simulink model "microphone_PDM"  (R2016b)
settings: Solver=ode5  StartTime=0.0  StopTime=2*pi*200000/2.4e6  MaxStep=1/512000  RelTol=1e-3  AbsTol=1e-6
PreLoadFcn:
  | input_rate = 2.5e6;
  | input_period = 1/input_rate;
  | decimation_factor = 64;
  | 
  | 
  | ila_PDM_data = read_vectored_ILA_PDM_capture('.\ILA_capture\iladata_A440_vectors_1024.csv');
  | % ila_PDM_data = read_vectored_ILA_PDM_capture('.\ILA_capture\iladata_speech_vectors_1024.csv');
  | 
  | ila_data_struct.time = [];
  | ila_data_struct.signals.values = ila_PDM_data;
StopFcn:
  | p = audioplayer(squeeze(simout_sysgen_PCM_audio.Data), input_rate/decimation_factor);
  | play(p, [1 (get(p, 'SampleRate') * 1)]);
  | 
  | % p = audioplayer(squeeze(simout_floating_point_PCM_audio.Data), input_rate/decimation_factor);
  | % play(p, [1 (get(p, 'SampleRate') * 1)]);
undefined symbols (not defined in the file): xlfda_numerator
libraries: xbsIndex_r4 x17, dspmlti4 x2, simulink x1, dspmisc x1
settings Model: ExtModeTrigMode=oneshot  ExtModeArmWhenConnect=off  ExtModeAutoUpdateStatusClock=off  Creator=The MathWorks Inc.  LastModifiedBy=Luc
settings DataIOCC: SaveFormat=Array  SaveOutput=off  SaveTime=off  SignalLoggingName=logsOut
settings OptimizationCC: BlockReduction=off  BooleanDataType=off  ExpressionDepthLimit=2147483647  RollThreshold=2  InitFltsAndDblsToZero=on  EfficientMapNaN2IntZero=off  LifeSpan=inf
settings DebuggingCC: SaveWithParameterizedLinksMsg=none  UnderspecifiedInitializationDetection=Classic  MergeDetectMultiDrivingBlocksExec=none  SignalResolutionControl=TryResolveAllWithWarning  MultiTaskDSMMsg=warning  MultiTaskCondExecSysMsg=none  IntegerOverflowMsg=none  FcnCallInpInsideContextMsg=warning  StateNameClashWarn=warning  SFUnexpectedBacktrackingDiag=warning  SFNoUnconditionalDefaultTransitionDiag=warning  SFExecutionAtInitializationDiag=none  IntegerSaturationMsg=none
settings HardwareCC: ProdBitPerPointer=32  ProdBitPerSizeT=32  ProdBitPerPtrDiffT=32  ProdLargestAtomicFloat=None  ProdIntDivRoundTo=Undefined  ProdEndianess=Unspecified  ProdWordSize=32  ProdHWDeviceType=32-bit Generic  TargetUnknown=on
settings ModelReferenceCC: PropagateSignalLabelsOutOfModel=off
settings GRTTargetCC: TargetFcnLib=ansi_tfl_tmw.mat  TargetLangStandard=C89/C90 (ANSI)  GeneratePreprocessorConditionals=Disable all  CombineOutputUpdateFcns=off  GRTInterface=on
settings ConfigComp: CovMetricSettings=dw  CovHtmlReporting=on  CovSaveCumulativeToWorkspaceVar=on  CovSaveSingleToWorkspaceVar=on  CovExternalEMLEnable=off

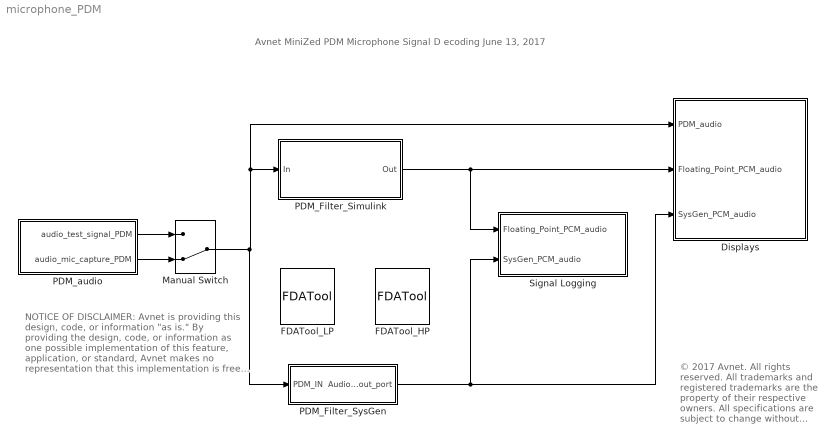
== system microphone_PDM ==
  note: Avnet MiniZed PDM Microphone Signal D ecoding
      | June 13, 2017
  note: NOTICE OF DISCLAIMER: Avnet is providing this design, code, or information "as is." By providing the design, code, or information as one possible implementation of this feature, application, or standard, Avnet makes no representation that this implementation is free from any claims of infringement. You are responsible for obtaining any rights you may require for your implementation. Avnet expressly disclaims any warranty whatsoever with respect to the adequacy of the implementation, including but not limited to any warranties or representations that this implementation is free from claims of infringement and any implied warranties of merchantability or fitness for a particular purpose.
  note: © 2017 Avnet. All rights reserved. All trademarks and registered trademarks are the property of their respective owners. All specifications are subject to change without notice.
  Displays : Subsystem
  FDATool_HP : xbsIndex_r4/FDATool  block_type=fdatool
      settings: infoedit=FDATool
  FDATool_LP : xbsIndex_r4/FDATool  block_type=fdatool
      settings: infoedit=FDATool
  Manual Switch : ManualSwitch  CurrentSetting=0
  PDM_Filter_Simulink : Subsystem
  PDM_Filter_SysGen : Subsystem
      mask Display: image('Avnet_Reach_Further_2017_green.png');
  PDM_audio : Subsystem
  Signal Logging : Subsystem
  wires:
  PDM_Filter_SysGen/1(Audio_out_port) -> Displays/3(SysGen_PCM_audio), Signal Logging/2(SysGen_PCM_audio)
  PDM_Filter_Simulink/1(Out) -> Signal Logging/1(Floating_Point_PCM_audio), Displays/2(Floating_Point_PCM_audio)
  PDM_audio/2(audio_mic_capture_PDM) -> Manual Switch/2
  PDM_audio/1(audio_test_signal_PDM) -> Manual Switch/1
  Manual Switch/1 -> PDM_Filter_SysGen/1(PDM_IN), Displays/1(PDM_audio), PDM_Filter_Simulink/1(In)

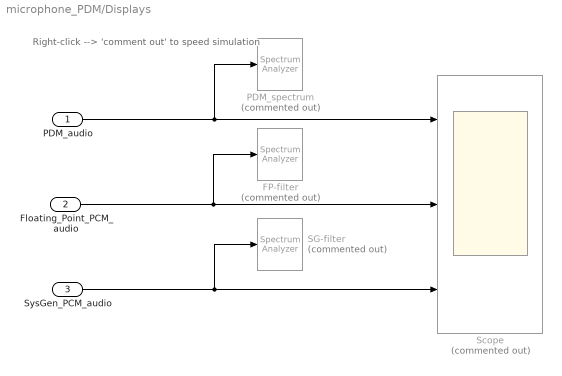
== system microphone_PDM/Displays ==
  note: Right-click --> 'comment out' to speed simulation
  PDM_audio : Inport
  Floating_Point_PCM_audio : Inport  Port=2
  SysGen_PCM_audio : Inport  Port=3
  FP-filter : SpectrumAnalyzer  Commented=on
  PDM_spectrum : SpectrumAnalyzer  Commented=on
  SG-filter : SpectrumAnalyzer  Commented=on
  Scope : Scope  Commented=on  NumInputPorts=3
  wires:
  SysGen_PCM_audio/1 -> SG-filter/1, Scope/3
  PDM_audio/1 -> PDM_spectrum/1, Scope/1
  Floating_Point_PCM_audio/1 -> FP-filter/1, Scope/2

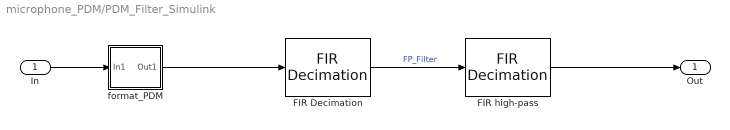
== system microphone_PDM/PDM_Filter_Simulink ==
  In : Inport
  FIR Decimation : dspmlti4/FIR Decimation  FilterSource=Dialog parameters  h=xlfda_numerator([bdroot '/FDATool_LP'])  D=decimation_factor  filtStruct=Direct form  FilterObject=Hm_firdecim  InputProcessing=Columns as channels (frame based)  framing=Allow multirate processing  inputOffset=0  outputBufInitCond=0  roundingMode=Floor  overflowMode=off  firstCoeffDataTypeStr=Inherit: Same word length as input  firstCoeffMin=[]  firstCoeffMax=[]  firstCoeffLastDataTypeStr=Inherit: Same word length as input  outputDataTypeStr=Inherit: Same as accumulator  outputMin=[]  outputMax=[]  outputLastDataTypeStr=Inherit: Same as accumulator
  "FIR high-pass " : dspmlti4/FIR Decimation  FilterSource=Dialog parameters  h=xlfda_numerator([bdroot '/FDATool_HP'])  D=1  filtStruct=Direct form  FilterObject=Hm_firdecim  InputProcessing=Columns as channels (frame based)  framing=Allow multirate processing  inputOffset=0  outputBufInitCond=0  roundingMode=Floor  overflowMode=off  firstCoeffDataTypeStr=Inherit: Same word length as input  firstCoeffMin=[]  firstCoeffMax=[]  firstCoeffLastDataTypeStr=Inherit: Same word length as input  outputDataTypeStr=Inherit: Same as accumulator  outputMin=[]  outputMax=[]  outputLastDataTypeStr=Inherit: Same as accumulator
  format_PDM : Subsystem
  Out : Outport
  wires:
  FIR Decimation/1 -> "FIR high-pass "/1  "FP_Filter"
  In/1 -> format_PDM/1(In1)
  "FIR high-pass "/1 -> Out/1
  format_PDM/1(Out1) -> FIR Decimation/1

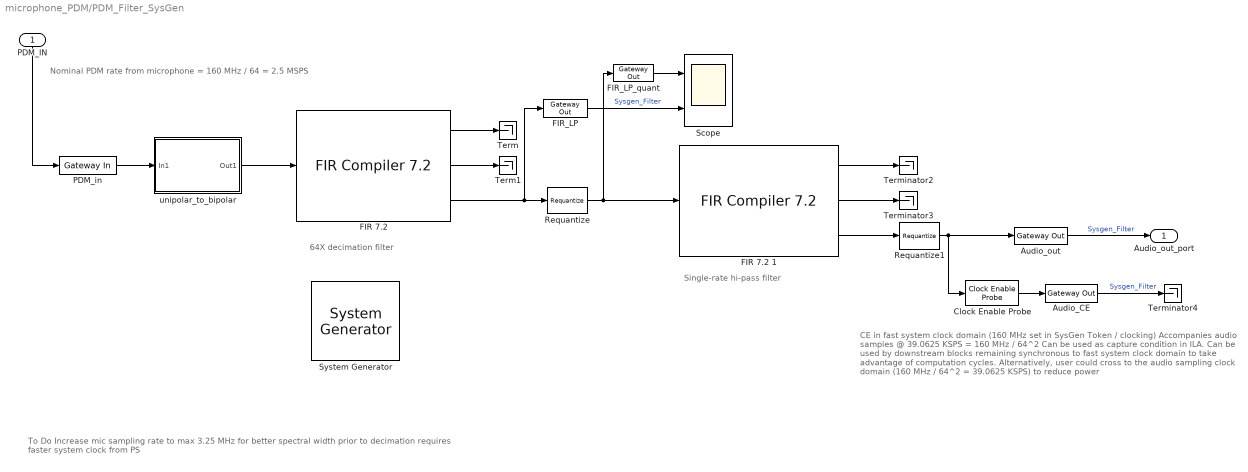
== system microphone_PDM/PDM_Filter_SysGen ==
  note: CE in fast system clock domain (160 MHz set in SysGen Token / clocking)
      | Accompanies audio samples @ 39.0625 KSPS = 160 MHz / 64^2
      |
      | Can be used as capture condition in ILA.
      |
      | Can be used by downstream blocks remaining synchronous to fast system clock domain to take advantage of computation cycles.
      |
      | Alternatively, user could cross to the audio sampling clock domain (160 MHz / 64^2 = 39.0625 KSPS) to reduce power
  note: Nominal PDM rate from microphone = 160 MHz / 64 = 2.5 MSPS
  note: 64X decimation filter
  note: Single-rate hi-pass filter
  note: To Do
      |
      | Increase mic sampling rate to max 3.25 MHz for better spectral width prior to decimation
      | requires faster system clock from PS
  PDM_IN : Inport
  " System Generator" : xbsIndex_r4/ System Generator  Tag=genX  xilinxfamily=zynq  part=xc7z007s  speed=-1  package=clg225  synthesis_tool=Vivado  clock_wrapper=Clock Enables  directory=C:/des/AvnetGIT/hdl/IP/PDM_Filter  proj_type=Vivado  Synth_file=Vivado Synthesis Defaults  Impl_file=Vivado Implementation Defaults  testbench=off  simulink_period=1/(64*2.5e6)  sysclk_period=6.25  dcm_input_clock_period=10  incr_netlist=off  trim_vbits=Everywhere in SubSystem  dbl_ovrd=According to Block Masks  core_generation=According to Block Masks  run_coregen=off  deprecated_control=off  eval_field=0  block_type=sysgen
  Audio_CE : xbsIndex_r4/Gateway Out  inherit_from_input=off  hdl_port=on  rows=1  columns=1  UseAsDAC=off  DACChannel='1'  interface=None  automatic_assignment=on  address_offset=hex2dec('00')  intf_name=''  intf_description=''  timing_constraint=None  locs_specified=off  LOCs={}  io_standard={}  block_type=gatewayout
  Audio_out : xbsIndex_r4/Gateway Out  inherit_from_input=off  hdl_port=on  rows=1  columns=1  UseAsDAC=off  DACChannel='1'  interface=None  automatic_assignment=on  address_offset=hex2dec('00')  intf_name=''  intf_description=''  timing_constraint=None  locs_specified=off  LOCs={}  io_standard={}  block_type=gatewayout
  Clock Enable Probe : xbsIndex_r4/Clock Enable Probe  inherit_constraints=off  block_type=ceprobe
      settings: infoedit="Clock enable extractor.  Produces a Boolean output that mirrors the hardware clock enable associated with the input sample rate.<br><br>Hardware notes: in hardware this block costs nothing."
  "FIR 7.2 " : xbsIndex_r4/FIR Compiler 7.2   coefficientvector=xlfda_numerator([bdroot '/FDATool_LP'])* decimation_factor  coefficient_sets=1  coefficient_reload=off  filter_type=Decimation  rate_change_type=Integer  interpolation_rate=1  decimation_rate=decimation_factor  zero_pack_factor=1  channel_sequence=Basic  number_channels=1  pattern_list='P4-0,P4-1,P4-2,P4-3,P4-4'  number_paths=1  ratespecification=Maximum_Possible  sampleperiod=4096  hardwareoversamplingrate=1  coefficient_sign=Signed  quantization=Maximize_Dynamic_Range  coefficient_width=16  bestprecision=on  coefficient_fractional_bits=15  coefficient_structure=Symmetric  output_rounding_mode=Symmetric_Rounding_to_Infinity  output_width=21  filter_architecture=Systolic_Multiply_Accumulate  optimization_goal=Area  optimization_list='None'  data_buffer_type=Automatic  coefficient_buffer_type=Automatic  input_buffer_type=Automatic  output_buffer_type=Automatic  preference_for_other_storage=Automatic  multi_column_support=Automatic  columnconfig='10'  inter_column_pipe_length=4  data_has_tlast=Not_Required  m_data_has_tready=off  s_data_has_fifo=off  s_data_has_tuser=Not_Required  m_data_has_tuser=Not_Required  s_config_sync_mode=On_Vector  s_config_method=Single  num_reload_slots=1  has_aclken=off  has_aresetn=off  infoeditControl=ARESETn must be asserted for a minimum of 2 cycles  reset_data_vector=on  trim_axipin_name=on  simulation_type=hybrid_sim  simulation_model=sysgen:xfirv7_2_cmodel  data_path_portlist={ 's_axis_data_tdata', 'm_axis_data_tdata' }  passband_min=0.0  passband_max=0.5  stopband_min=0.5  stopband_max=1.0  filter_selection=1  gui_behaviour='Sysgen_GUI'  data_sign=Signed  data_width=16  data_fractional_bits=0  data_tuser_width=1  wrapper_available=true  ip_wrap_arbitrary_binary_point=true  ip_name=FIR Compiler  ip_version=7.2  dsptool_ready=true  ipcore_usecache=true  ipcore_useipmodelcache=true  port_translation_map={ 'aclken' => 'en', 'aresetn' => 'rst' }  run_core_at_system_period=true  ipcore_xco_need_fpga_part=true  block_type=fir_compiler_v7_2
      settings: infoedit=Maximum Possible : Maximizes oversampling rate. Abstracted input handshake (no s_data_tvalid) and automatic rate propagation.<br>Hardware Oversampling Rate : Specifies oversampling rate relative to the input sample period. Abstracted input handshake (no s_data_tvalid) and automatic rate propagation.<br>Input/Output Sample Period : Specifies absolute oversampling rate. No input handshake abstraction (exposes s_data_tvalid) and no rate propagation.
  FIR 7.2 1 : xbsIndex_r4/FIR Compiler 7.2   coefficientvector=xlfda_numerator([bdroot '/FDATool_HP'])  coefficient_sets=1  coefficient_reload=off  filter_type=Single_Rate  rate_change_type=Integer  interpolation_rate=1  decimation_rate=1  zero_pack_factor=1  channel_sequence=Basic  number_channels=1  pattern_list='P4-0,P4-1,P4-2,P4-3,P4-4'  number_paths=1  ratespecification=Maximum_Possible  sampleperiod=1  hardwareoversamplingrate=1  coefficient_sign=Signed  quantization=Maximize_Dynamic_Range  coefficient_width=16  bestprecision=on  coefficient_fractional_bits=15  coefficient_structure=Symmetric  output_rounding_mode=Symmetric_Rounding_to_Infinity  output_width=16  filter_architecture=Systolic_Multiply_Accumulate  optimization_goal=Area  optimization_list='None'  data_buffer_type=Automatic  coefficient_buffer_type=Automatic  input_buffer_type=Automatic  output_buffer_type=Automatic  preference_for_other_storage=Automatic  multi_column_support=Automatic  columnconfig='40,40'  inter_column_pipe_length=4  data_has_tlast=Not_Required  m_data_has_tready=off  s_data_has_fifo=off  s_data_has_tuser=Not_Required  m_data_has_tuser=Not_Required  s_config_sync_mode=On_Vector  s_config_method=Single  num_reload_slots=1  has_aclken=off  has_aresetn=off  infoeditControl=ARESETn must be asserted for a minimum of 2 cycles  reset_data_vector=on  trim_axipin_name=on  simulation_type=hybrid_sim  simulation_model=sysgen:xfirv7_2_cmodel  data_path_portlist={ 's_axis_data_tdata', 'm_axis_data_tdata' }  passband_min=0.0  passband_max=0.5  stopband_min=0.5  stopband_max=1.0  filter_selection=1  gui_behaviour='Sysgen_GUI'  data_sign=Signed  data_width=16  data_fractional_bits=0  data_tuser_width=1  wrapper_available=true  ip_wrap_arbitrary_binary_point=true  ip_name=FIR Compiler  ip_version=7.2  dsptool_ready=true  ipcore_usecache=true  ipcore_useipmodelcache=true  port_translation_map={ 'aclken' => 'en', 'aresetn' => 'rst' }  run_core_at_system_period=true  ipcore_xco_need_fpga_part=true  block_type=fir_compiler_v7_2
      settings: infoedit=Maximum Possible : Maximizes oversampling rate. Abstracted input handshake (no s_data_tvalid) and automatic rate propagation.<br>Hardware Oversampling Rate : Specifies oversampling rate relative to the input sample period. Abstracted input handshake (no s_data_tvalid) and automatic rate propagation.<br>Input/Output Sample Period : Specifies absolute oversampling rate. No input handshake abstraction (exposes s_data_tvalid) and no rate propagation.
  FIR_LP : xbsIndex_r4/Gateway Out  inherit_from_input=off  hdl_port=off  rows=1  columns=1  UseAsDAC=off  DACChannel='1'  interface=None  automatic_assignment=on  address_offset=hex2dec('00')  intf_name=''  intf_description=''  timing_constraint=None  locs_specified=off  LOCs={}  io_standard={}  block_type=gatewayout
  FIR_LP_quant : xbsIndex_r4/Gateway Out  inherit_from_input=off  hdl_port=off  rows=1  columns=1  UseAsDAC=off  DACChannel='1'  interface=None  automatic_assignment=on  address_offset=hex2dec('00')  intf_name=''  intf_description=''  timing_constraint=None  locs_specified=off  LOCs={}  io_standard={}  block_type=gatewayout
  PDM_in : xbsIndex_r4/Gateway In  gui_display_data_type=Boolean  arith_type=Boolean  n_bits=1  bin_pt=0  preci_type=Single  exp_width=8  frac_width=24  rows=1  columns=1  quantization=Truncate  overflow=Flag as error  period=1/input_rate  UseAsADC=off  ADCChannel='1'  interface=None  automatic_assignment=on  address_offset=hex2dec('00')  intf_name=''  intf_description=''  default_value=0  timing_constraint=None  locs_specified=off  LOCs={}  io_standard={}  inherit_from_input=off  hdl_port=on  dbl_ovrd=off  block_type=gatewayin
  Requantize : xbsIndex_r4/Requantize  scale_factor=0  n_bits=14  bin_pt=11  simulation_type=fast_sim  simulation_model=sysgen:requantizer  block_type=requantizer
  Requantize1 : xbsIndex_r4/Requantize  scale_factor=0  n_bits=16  bin_pt=13  simulation_type=fast_sim  simulation_model=sysgen:requantizer  block_type=requantizer
  Scope : Scope  NumInputPorts=2
  Term : Terminator
  Term1 : Terminator
  Terminator2 : Terminator
  Terminator3 : Terminator
  Terminator4 : Terminator
  unipolar_to_bipolar : Subsystem
  Audio_out_port : Outport
  wires:
  Audio_out/1 -> Audio_out_port/1  "Sysgen_Filter"
  "FIR 7.2 "/1 -> Term/1
  "FIR 7.2 "/2 -> Term1/1
  PDM_IN/1 -> PDM_in/1
  PDM_in/1 -> unipolar_to_bipolar/1(In1)
  "FIR 7.2 "/3 -> FIR_LP/1, Requantize/1
  FIR 7.2 1/1 -> Terminator2/1
  FIR 7.2 1/2 -> Terminator3/1
  FIR 7.2 1/3 -> Requantize1/1
  Clock Enable Probe/1 -> Audio_CE/1
  Audio_CE/1 -> Terminator4/1  "Sysgen_Filter"
  unipolar_to_bipolar/1(Out1) -> "FIR 7.2 "/1
  Requantize/1 -> FIR_LP_quant/1, FIR 7.2 1/1
  Requantize1/1 -> Clock Enable Probe/1, Audio_out/1
  FIR_LP_quant/1 -> Scope/1
  FIR_LP/1 -> Scope/2  "Sysgen_Filter"

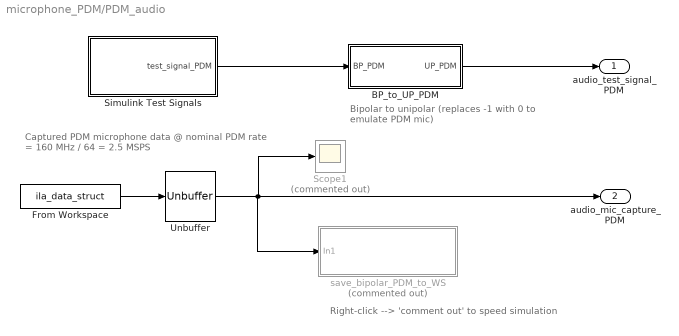
== system microphone_PDM/PDM_audio ==
  note: Bipolar to unipolar
      | (replaces -1 with 0 to emulate PDM mic)
  note: Right-click --> 'comment out' to speed simulation
  note: Captured PDM microphone data @ nominal PDM rate = 160 MHz / 64 = 2.5 MSPS
  BP_to_UP_PDM : Subsystem
  From Workspace : FromWorkspace  VariableName=ila_data_struct  OutDataTypeStr=double  SampleTime=input_period*1024  Interpolate=off  OutputAfterFinalValue=Cyclic repetition
  Scope1 : Scope  Commented=on
  Simulink Test Signals : Subsystem  mask{audio_tone_freq=440, sub_audio_freq=5}
      mask prompts: audio_tone_freq "Audio tone frequency (Hz)"; sub_audio_freq "sub audio noise freq (Hz)"
  Unbuffer : Unbuffer  SampleBasedProcessing=Same as frame based
  save_bipolar_PDM_to_WS : Subsystem  Commented=on
  audio_test_signal_PDM : Outport
  audio_mic_capture_PDM : Outport  Port=2
  wires:
  BP_to_UP_PDM/1(UP_PDM) -> audio_test_signal_PDM/1
  From Workspace/1 -> Unbuffer/1
  Unbuffer/1 -> save_bipolar_PDM_to_WS/1(In1), audio_mic_capture_PDM/1, Scope1/1
  Simulink Test Signals/1(test_signal_PDM) -> BP_to_UP_PDM/1(BP_PDM)

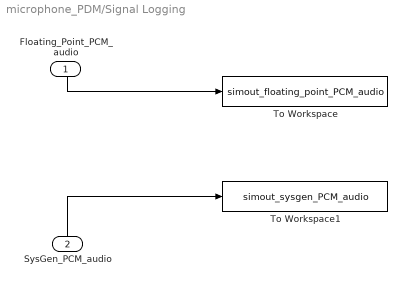
== system microphone_PDM/Signal Logging ==
  Floating_Point_PCM_audio : Inport
  SysGen_PCM_audio : Inport  Port=2
  To Workspace : ToWorkspace  VariableName=simout_floating_point_PCM_audio  SaveFormat=Timeseries  SampleTime=-1
  To Workspace1 : ToWorkspace  VariableName=simout_sysgen_PCM_audio  SaveFormat=Timeseries  SampleTime=-1
  wires:
  SysGen_PCM_audio/1 -> To Workspace1/1
  Floating_Point_PCM_audio/1 -> To Workspace/1

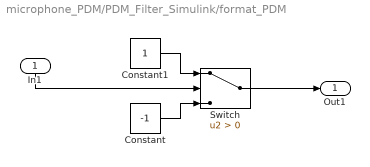
== system microphone_PDM/PDM_Filter_Simulink/format_PDM ==
  In1 : Inport
  Constant : Constant  Value=-1
  Constant1 : Constant
  Switch : Switch  Criteria=u2 > Threshold
  Out1 : Outport
  wires:
  In1/1 -> Switch/2
  Constant1/1 -> Switch/1
  Constant/1 -> Switch/3
  Switch/1 -> Out1/1

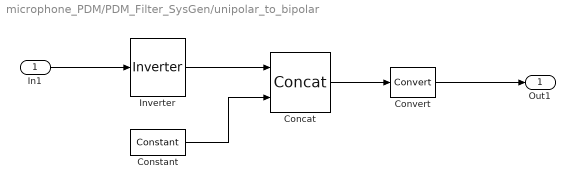
== system microphone_PDM/PDM_Filter_SysGen/unipolar_to_bipolar ==
  In1 : Inport
  Concat : xbsIndex_r4/Concat  num_inputs=2  dbl_ovrd=off  block_type=concat
  Constant : xbsIndex_r4/Constant  const=1.0  gui_display_data_type=Boolean  arith_type=Boolean  n_bits=16  bin_pt=14  preci_type=Single  exp_width=8  frac_width=24  explicit_period=off  period=1  equ=P=C  opselect=C  inp2=PCIN>>17  opr=+  inp1=P  carry=CIN  dbl_ovrd=off  block_type=constant
  Convert : xbsIndex_r4/Convert  gui_display_data_type=Fixed-point  arith_type="Signed  (2's comp)"  n_bits=2  bin_pt=0  float_type=Single  exp_bits=8  fraction_bits=24  quantization=Truncate  overflow=Wrap  en=off  latency=1  pipeline=off  dbl_ovrd=off  block_type=convert
  Inverter : xbsIndex_r4/Inverter  en=off  latency=1  dbl_ovrd=off  block_type=inv
  Out1 : Outport
  wires:
  Constant/1 -> Concat/2
  Inverter/1 -> Concat/1
  In1/1 -> Inverter/1
  Convert/1 -> Out1/1
  Concat/1 -> Convert/1

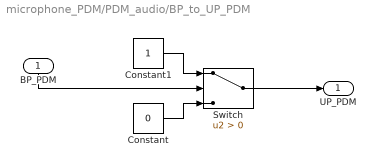
== system microphone_PDM/PDM_audio/BP_to_UP_PDM ==
  BP_PDM : Inport
  Constant : Constant  Value=0
  Constant1 : Constant
  Switch : Switch  Criteria=u2 > Threshold
  UP_PDM : Outport
  wires:
  BP_PDM/1 -> Switch/2
  Constant1/1 -> Switch/1
  Constant/1 -> Switch/3
  Switch/1 -> UP_PDM/1

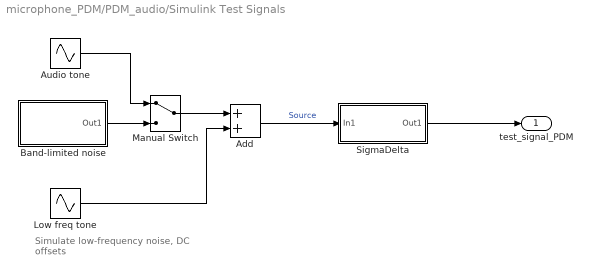
== system microphone_PDM/PDM_audio/Simulink Test Signals ==
  note: Simulate low-frequency noise, DC offsets
  Add : Sum
  Audio tone : Sin  Amplitude=0.5  Frequency=2*pi*audio_tone_freq  SampleTime=input_period
  Band-limited noise : Subsystem
  Low freq tone : Sin  Amplitude=0.0  Frequency=2*pi*sub_audio_freq  SampleTime=input_period
  Manual Switch : ManualSwitch
  SigmaDelta : Subsystem
  test_signal_PDM : Outport
  wires:
  Add/1 -> SigmaDelta/1(In1)  "Source"
  Low freq tone/1 -> Add/2
  Manual Switch/1 -> Add/1
  Audio tone/1 -> Manual Switch/1
  Band-limited noise/1(Out1) -> Manual Switch/2
  SigmaDelta/1(Out1) -> test_signal_PDM/1

== system microphone_PDM/PDM_audio/save_bipolar_PDM_to_WS ==
  note: Unipolar to Bipolar
      | (replaces 0 with -1)
  In1 : Inport
  To Workspace2 : ToWorkspace  VariableName=simout_captured_data_PDM_bipolar  SaveFormat=Timeseries  SampleTime=-1
  format_PDM1 : Subsystem
  wires:
  In1/1 -> format_PDM1/1(In1)
  format_PDM1/1(Out1) -> To Workspace2/1

== system microphone_PDM/PDM_audio/Simulink Test Signals/Band-limited noise ==
  Band-Limited White Noise : simulink/Sources/Band-Limited White Noise  Cov=[0.000001]  Ts=input_period  seed=[23341]
  Low pass Filter : DiscreteFir  Coefficients=xlfda_numerator([bdroot '/FDATool_LP'])
  Out1 : Outport
  wires:
  Band-Limited White Noise/1 -> Low pass Filter/1
  Low pass Filter/1 -> Out1/1

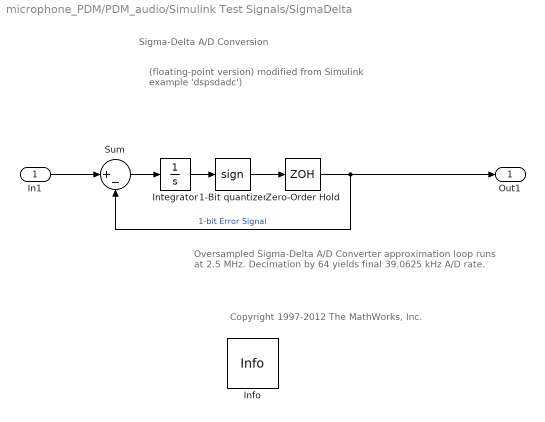
== system microphone_PDM/PDM_audio/Simulink Test Signals/SigmaDelta ==
  note: Oversampled Sigma-Delta A/D Converter
      | approximation loop runs at 2.5 MHz.
      | Decimation by 64 yields final 39.0625 kHz A/D rate.
  note: Copyright 1997-2012 The MathWorks, Inc.
  note: Sigma-Delta A/D Conversion
  note: (floating-point version)
      | modified from Simulink example 'dspsdadc')
  In1 : Inport
  1-Bit quantizer : Signum
  Info : dspmisc/Info  SystemSampleTime=-1
  Integrator : Integrator
  Sum : Sum  Inputs=|+-  SaturateOnIntegerOverflow=on  InputSameDT=on  OutDataTypeStr=Inherit: Same as first input
  Zero-Order Hold : ZeroOrderHold  SampleTime=input_period
  Out1 : Outport
  wires:
  Zero-Order Hold/1 -> Out1/1, Sum/2  "1-bit Error Signal"
  1-Bit quantizer/1 -> Zero-Order Hold/1
  Sum/1 -> Integrator/1
  Integrator/1 -> 1-Bit quantizer/1
  In1/1 -> Sum/1

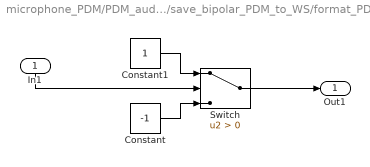
== system microphone_PDM/PDM_audio/save_bipolar_PDM_to_WS/format_PDM1 ==
  In1 : Inport
  Constant : Constant  Value=-1
  Constant1 : Constant
  Switch : Switch  Criteria=u2 > Threshold
  Out1 : Outport
  wires:
  In1/1 -> Switch/2
  Constant1/1 -> Switch/1
  Constant/1 -> Switch/3
  Switch/1 -> Out1/1
